simulink model "myPIDmodel"  (R2023a)
settings: Solver=FixedStepAuto  StartTime=0.0  StopTime=10.0  FixedStep=.01  RelTol=1e-3
undefined symbols (not defined in the file or in its folder): DiscIntNeverNeededParam
libraries: simulink x1
settings Model: Creator=Sam  LastModifiedBy=Sam

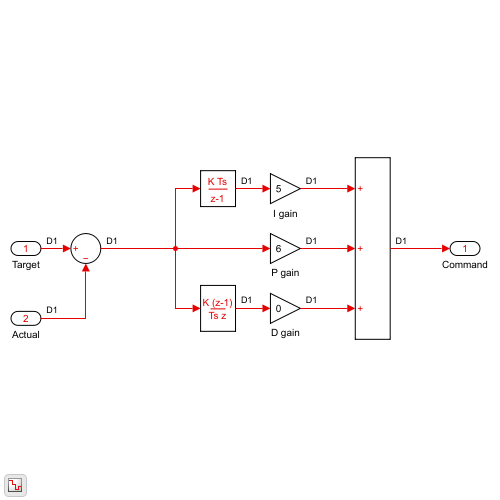
[thumbnail: Simulink's stored preview of the top-level diagram]
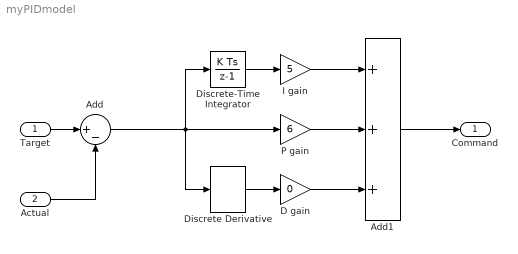
== system myPIDmodel ==
  Target : Inport  PortDimensions=[1]  SampleTime=.01
  Actual : Inport  Port=2  PortDimensions=[1]  SampleTime=.01
  Add : Sum  Inputs=|+-
  Add1 : Sum  Inputs=+++
  D gain : Gain  Gain=0
  Discrete Derivative : simulink/Discrete/Discrete Derivative  gainval=1.0  ICPrevScaledInput=0.0  OutMin=[]  OutMax=[]  OutDataType=fixdt(1, 16)  OutScaling=2^-10  DoSatur=off
  Discrete-Time Integrator : DiscreteIntegrator  SampleTime=-1  ICPrevOutput=DiscIntNeverNeededParam  ICPrevScaledInput=DiscIntNeverNeededParam
  I gain : Gain  Gain=5
  P gain : Gain  Gain=6
  Command : Outport  SampleTime=.01
  wires:
  Add/1 -> Discrete Derivative/1, Discrete-Time Integrator/1, P gain/1
  Discrete-Time Integrator/1 -> I gain/1
  Target/1 -> Add/1
  Actual/1 -> Add/2
  Discrete Derivative/1 -> D gain/1
  P gain/1 -> Add1/2
  I gain/1 -> Add1/1
  D gain/1 -> Add1/3
  Add1/1 -> Command/1
